simulink model "slexPowerWindowControl"  (R2014b)
settings: Solver=ode23  StartTime=0  StopTime=10  FixedStep=1e-4  RelTol=1e-3
Description:
  | Power Window Controller
settings Model: Creator=The MathWorks Inc.  LastModifiedBy=The MathWorks Inc.
settings DataIOCC: LimitDataPoints=off  SaveCompleteFinalSimState=on  SaveState=on  SignalLoggingName=sigsOut
settings OptimizationCC: InlineParams=on  ExpressionDepthLimit=2147483647
settings DebuggingCC: UnderspecifiedInitializationDetection=Classic  MergeDetectMultiDrivingBlocksExec=none  SolverPrmCheckMsg=none  MultiTaskDSMMsg=warning  SigSpecEnsureSampleTimeMsg=none  FcnCallInpInsideContextMsg=UseLocalSettings  StateNameClashWarn=warning

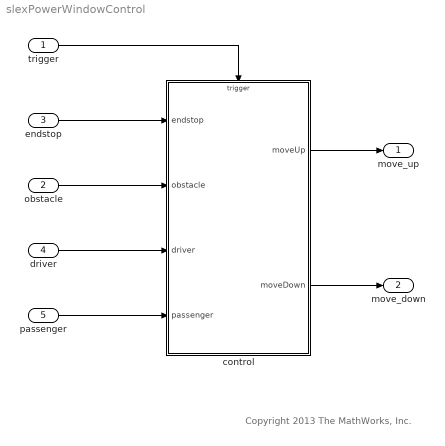
== system slexPowerWindowControl ==
  note: Copyright 2013 The MathWorks, Inc.
  trigger : Inport  OutDataTypeStr=double  SampleTime=0.01
  obstacle : Inport  Port=2  OutDataTypeStr=boolean
  endstop : Inport  Port=3  OutDataTypeStr=boolean
  driver : Inport  Port=4  OutDataTypeStr=boolean
  passenger : Inport  Port=5  OutDataTypeStr=boolean
  control : Stateflow chart  TreatAsAtomicUnit=on
  move_up : Outport  OutDataTypeStr=boolean
  move_down : Outport  Port=2  OutDataTypeStr=boolean
  wires:
  control/2(moveDown) -> move_down/1
  control/1(moveUp) -> move_up/1
  endstop/1 -> control/1(endstop)
  obstacle/1 -> control/2(obstacle)
  driver/1 -> control/3(driver)
  passenger/1 -> control/4(passenger)
  trigger/1 -> control/Trigger

== stateflow chart slexPowerWindowControl/control ==
  settings: executeAtInitialization=1
  state safe
    state driverNeutral
      entry:
      moveUp = 0;
      moveDown = 0;
      state passengerneutral
        entry:
        moveUp = 0;
        moveDown = 0;
      state passengerDown
        entry: moveDown = 1;
        exit: moveDown = 0;
        state iniPassengerDown
        state passengerDown
        state autoPassengerDown
        iniPassengerDown -> (junction 54) : after(100,ticks)
        (junction 54) -> autoPassengerDown [order 1] : [passenger[1]]
        (junction 54) -> safe.driverNeutral.passengerDown.passengerDown [order 2]
      state passengerUp
        entry: moveUp = 1;
        exit: moveUp = 0;
        state iniPassengerUp
        state PassengerUp
        state autoPassengerUp
        iniPassengerUp -> (junction 55) : after(100,ticks)
        (junction 55) -> PassengerUp [order 2]
        (junction 55) -> autoPassengerUp [order 1] : [passenger[1]]
      (default) -> passengerneutral
      passengerneutral -> iniPassengerUp [order 1] : [passenger[2]]
      passengerneutral -> iniPassengerDown [order 2] : [passenger[3]]
      safe.driverNeutral.passengerDown.passengerDown -> passengerneutral : [passenger[1]]
      safe.driverNeutral.passengerDown -> passengerneutral [order 1] : [endstop]
      PassengerUp -> passengerneutral : [passenger[1]]
      passengerUp -> passengerneutral [order 2] : [endstop]
      safe.driverNeutral.passengerDown -> PassengerUp [order 2] : [passenger[2]]
      passengerUp -> safe.driverNeutral.passengerDown.passengerDown [order 1] : [passenger[3]]
    state driverDown
      entry: moveDown = 1;
      exit: moveDown = 0;
      state iniDriverDown
      state autoDriverDown
      state DriverDown
      iniDriverDown -> (junction 56) : after(100,ticks)
      (junction 56) -> autoDriverDown [order 1] : [driver[1]]
      (junction 56) -> DriverDown [order 2]
    state driverUp
      entry: moveUp = 1;
      exit: moveUp = 0;
      state iniDriverUp
      state DriverUp
      state autoDriverUp
      iniDriverUp -> (junction 57) : after(100,ticks)
      (junction 57) -> DriverUp [order 2]
      (junction 57) -> autoDriverUp [order 1] : [driver[1]]
    (default) -> driverNeutral
    driverNeutral -> iniDriverDown [order 2] : [driver[3]]
    DriverDown -> driverNeutral : [driver[1]]
    driverDown -> driverNeutral [order 1] : [endstop]
    DriverUp -> driverNeutral : [driver[1]]
    driverUp -> driverNeutral [order 2] : [endstop]
    driverNeutral -> iniDriverUp [order 1] : [driver[2]]
    driverDown -> DriverUp [order 2] : [driver[2]]
    driverUp -> DriverDown [order 1] : [driver[3]]
  state emergencyDown
    entry:
    moveUp = 0;
    moveDown = 1;
  emergencyDown -> passengerneutral : [endstop | after(100,ticks)]
  (default) -> safe
  safe -> emergencyDown : [obstacle]
  data: moveUp output boolean; moveDown output boolean; endstop input boolean; obstacle input boolean; driver input boolean size=3; passenger input boolean size=3
  events: ticks input EITHER_EDGE_EVENT
